simulink model "sampleModel1717"  (R2023a)
settings: Solver=VariableStepAuto  StartTime=0.0  StopTime=10.0  RelTol=1e-3
libraries: hdlsllib x4, simulink x2
settings Model: Creator=user1  LastModifiedBy=user1

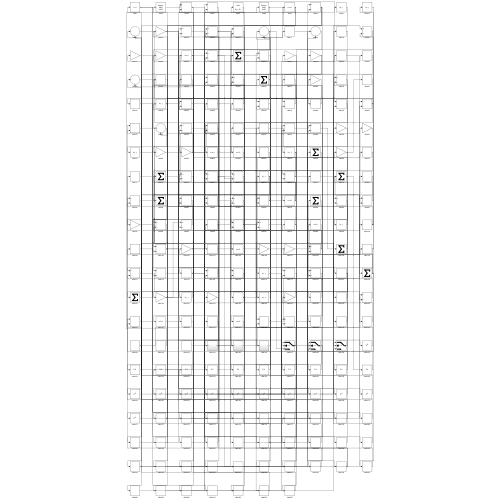
[thumbnail: Simulink's stored preview of the top-level diagram]
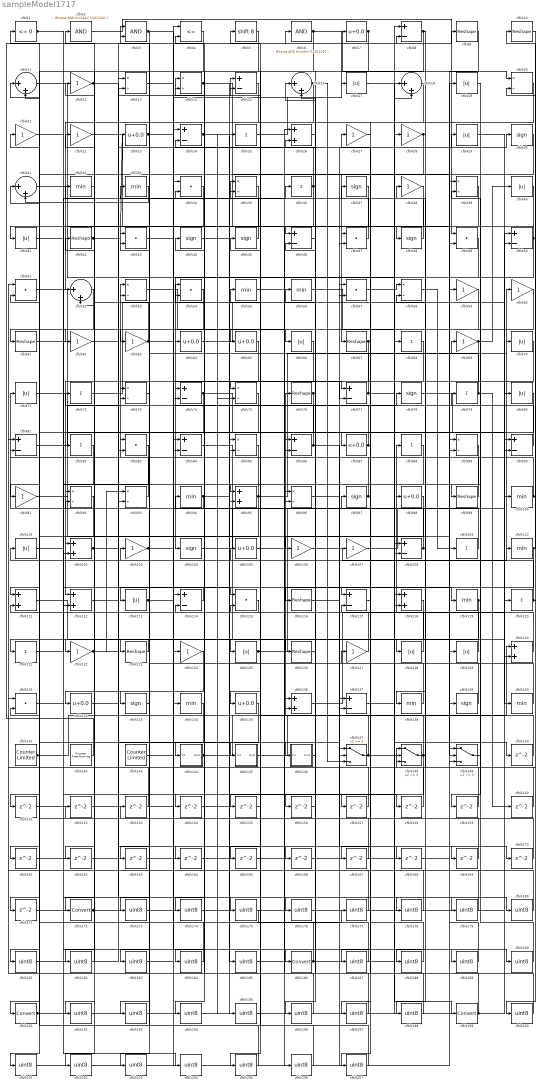
== system sampleModel1717 ==
  cfblk1 : hdlsllib/Logic and Bit Operations/Compare To Zero  relop=<=  OutDataTypeStr=boolean
  cfblk{9..10,42,61,67,76,99,116,123,126} (10 alike) : Reshape
  cfblk{32..33,55..56,94,100,110,119,134,138,140} (11 alike) : MinMax
  cfblk{17,19,29,40..41,66,70..71,80,101,113,125,128..129} (14 alike) : Abs  SaturateOnIntegerOverflow=off
  cfblk{26,95,102,111..112,118,130,136} (8 alike) : Sum
  cfblk{12,21..22,27..28,38,59..60,62..63,69,91,103,106..107,122,124,127} (18 alike) : Gain
  cfblk{30,37,44..45,48,78,97,104,133,139} (10 alike) : Signum
  cfblk{7,23,64..65,87,98,105,132,135} (9 alike) : Bias  Bias=0.0  SaturateOnIntegerOverflow=off
  cfblk{8,15,24,46,50,74,77,81,84,86,90,108,114,117,137} (15 alike) : Sum  Inputs=+-
  cfblk{25,36,68,72,79,82,88,109,120..121} (10 alike) : Sum  Inputs=+
  cfblk{11,16,18,31,52} (5 alike) : Sum  Inputs=|++
  cfblk{34,43,47,49,51,54,57,83,115,131} (10 alike) : DotProduct  OutDataTypeStr=Inherit: Inherit via internal rule
  cfblk{13..14,20,35,39,53,58,73,75,85,89,92..93,96} (14 alike) : Product  Inputs=*/  RndMeth=Zero  SaturateOnIntegerOverflow=on
  cfblk141 : hdlsllib/Sources/Counter Limited  uplimit=7  tsamp=-1
  cfblk142 : hdlsllib/Sources/Counter Free-Running  NumBits=16  tsamp=-1
  cfblk143 : hdlsllib/Sources/Counter Limited  uplimit=7  tsamp=-1
  cfblk144 : Subsystem
      settings: LibrarySourceBlock=|
      | hdlsllib/Ports &
      | Subsystems/Subsystem
  cfblk145 : Subsystem
      settings: LibrarySourceBlock=|
      | hdlsllib/Ports &
      | Subsystems/Subsystem
  cfblk146 : Subsystem
      settings: LibrarySourceBlock=|
      | hdlsllib/Ports &
      | Subsystems/Subsystem
  cfblk147 : Switch  SaturateOnIntegerOverflow=off  InputSameDT=off
  cfblk148 : Switch  SaturateOnIntegerOverflow=off  InputSameDT=off
  cfblk149 : Switch  SaturateOnIntegerOverflow=off  InputSameDT=off
  cfblk{150..171} (22 alike) : Delay  SampleTime=1
  cfblk{172,186,191,199} (4 alike) : DataTypeConversion  SaturateOnIntegerOverflow=off  RndMeth=Floor
  cfblk{173..185,187..190,192..198,200..207} (32 alike) : DataTypeConversion  OutDataTypeStr=uint8  SaturateOnIntegerOverflow=off  RndMeth=Floor
  cfblk2 : simulink/Logic and Bit Operations/Bitwise Operator  logicop=AND  UseBitMask=on  BitMask=bin2dec('11011001')  BitMaskRealWorld=Stored Integer
      settings: LibrarySourceBlock=|
      | hdlsllib/Logic and Bit
      | Operations/Bitwise
      | Operator
  cfblk3 : Logic  AllPortsSameDT=off  OutDataTypeStr=boolean
  cfblk4 : RelationalOperator  Operator=<=  OutDataTypeStr=boolean  InputSameDT=off
  cfblk5 : ArithShift  BitShiftNumber=8
  cfblk6 : simulink/Logic and Bit Operations/Bitwise Operator  logicop=AND  UseBitMask=on  BitMask=bin2dec('11011001')  BitMaskRealWorld=Stored Integer
      settings: LibrarySourceBlock=|
      | hdlsllib/Logic and Bit
      | Operations/Bitwise
      | Operator
  wires:
  cfblk58/1 -> cfblk109/1
  cfblk69/1 -> cfblk40/1, cfblk75/1
  cfblk86/1 -> cfblk53/1, cfblk158/1
  cfblk148/1 -> cfblk27/1, cfblk198/1, cfblk205/1
  cfblk109/1 -> cfblk71/1
  cfblk106/1 -> cfblk60/1
  cfblk49/1 -> cfblk104/1
  cfblk142/1 -> cfblk6/1
  cfblk66/1 -> cfblk112/1
  cfblk2/1 -> cfblk49/1
  cfblk10/1 -> cfblk148/1
  cfblk95/1 -> cfblk69/1, cfblk54/1, cfblk42/1, cfblk168/1, cfblk201/1
  cfblk28/1 -> cfblk67/1, cfblk61/1
  cfblk82/1 -> cfblk102/1
  cfblk123/1 -> cfblk121/1
  cfblk147/1 -> cfblk76/1, cfblk110/1
  cfblk128/1 -> cfblk88/1
  cfblk104/1 -> cfblk98/1
  cfblk130/1 -> cfblk37/1
  cfblk6/1 -> cfblk20/1, cfblk74/2
  cfblk51/1 -> cfblk114/1
  cfblk15/1 -> cfblk52/1
  cfblk72/1 -> cfblk50/1
  cfblk50/1 -> cfblk125/1, cfblk46/1
  cfblk114/1 -> cfblk113/1
  cfblk20/1 -> cfblk87/1
  cfblk61/1 -> cfblk84/2
  cfblk113/1 -> cfblk96/1, cfblk190/1
  cfblk65/1 -> cfblk74/1
  cfblk101/1 -> cfblk186/1
  cfblk141/1 -> cfblk130/1, cfblk1/1
  cfblk84/1 -> cfblk128/1
  cfblk32/1 -> cfblk52/2
  cfblk140/1 -> cfblk38/1
  cfblk81/1 -> cfblk73/1
  cfblk93/1 -> cfblk73/2
  cfblk22/1 -> cfblk48/1
  cfblk36/1 -> cfblk14/2, cfblk194/1
  cfblk125/1 -> cfblk97/1, cfblk155/1
  cfblk5/1 -> cfblk122/1
  cfblk59/1 -> cfblk64/1
  cfblk7/1 -> cfblk91/1, cfblk65/1
  cfblk14/1 -> cfblk89/1, cfblk146/1(In1)
  cfblk108/1 -> cfblk14/1, cfblk83/1
  cfblk30/1 -> cfblk123/1
  cfblk4/1 -> cfblk172/1
  cfblk127/1 -> cfblk5/1
  cfblk88/1 -> cfblk135/1
  cfblk60/1 -> cfblk66/1
  cfblk73/1 -> cfblk133/1
  cfblk47/1 -> cfblk35/1
  cfblk75/1 -> cfblk111/1
  cfblk34/1 -> cfblk41/1
  cfblk78/1 -> cfblk130/2
  cfblk76/1 -> cfblk132/1, cfblk174/1
  cfblk146/1(Out1) -> cfblk86/1
  cfblk27/1 -> cfblk117/1
  cfblk129/1 -> cfblk94/1
  cfblk103/1 -> cfblk78/1, cfblk9/1
  cfblk112/1 -> cfblk15/1
  cfblk110/1 -> cfblk20/2, cfblk112/2
  cfblk71/1 -> cfblk149/2
  cfblk25/1 -> cfblk7/1
  cfblk98/1 -> cfblk106/1
  cfblk11/1 -> cfblk47/1
  cfblk29/1 -> cfblk120/1
  cfblk19/1 -> cfblk99/1
  cfblk79/1 -> cfblk43/2, cfblk159/1, cfblk160/1
  cfblk137/1 -> cfblk199/1
  cfblk53/1 -> cfblk136/1
  cfblk67/1 -> cfblk77/2, cfblk187/1
  cfblk24/1 -> cfblk129/1, cfblk75/2
  cfblk149/1 -> cfblk79/1
  cfblk115/1 -> cfblk111/2
  cfblk33/1 -> cfblk31/2
  cfblk64/1 -> cfblk28/1
  cfblk136/1 -> cfblk90/1
  cfblk85/1 -> cfblk81/2
  cfblk74/1 -> cfblk118/2, cfblk83/2, cfblk195/1
  cfblk138/1 -> cfblk3/1
  cfblk105/1 -> cfblk119/1
  cfblk111/1 -> cfblk140/1
  cfblk119/1 -> cfblk171/1, cfblk203/1
  cfblk35/1 -> cfblk62/1
  cfblk77/1 -> cfblk15/2, cfblk70/1
  cfblk80/1 -> cfblk191/1
  cfblk45/1 -> cfblk24/2
  cfblk57/1 -> cfblk58/1
  cfblk42/1 -> cfblk23/1, cfblk22/1
  cfblk3/1 -> cfblk157/1, cfblk173/1
  cfblk63/1 -> cfblk17/1, cfblk32/1, cfblk77/1
  cfblk107/1 -> cfblk50/2
  cfblk122/1 -> cfblk8/2, cfblk93/1, cfblk30/1
  cfblk145/1(Out1) -> cfblk49/2
  cfblk139/1 -> cfblk105/1
  cfblk121/1 -> cfblk36/1
  cfblk94/1 -> cfblk25/1, cfblk92/2
  cfblk102/1 -> cfblk145/1(In1), cfblk166/1
  cfblk96/1 -> cfblk29/1
  cfblk83/1 -> cfblk102/2
  cfblk144/1(Out1) -> cfblk107/1, cfblk170/1
  cfblk16/1 -> cfblk63/1, cfblk93/2, cfblk147/3
  cfblk56/1 -> cfblk108/1
  cfblk62/1 -> cfblk126/1
  cfblk31/1 -> cfblk118/1
  cfblk97/1 -> cfblk44/1, cfblk197/1
  cfblk48/1 -> cfblk33/1
  cfblk87/1 -> cfblk2/1, cfblk54/2, cfblk56/1
  cfblk100/1 -> cfblk10/1, cfblk46/2
  cfblk9/1 -> cfblk89/2
  cfblk37/1 -> cfblk82/1
  cfblk99/1 -> cfblk72/1
  cfblk126/1 -> cfblk16/2
  cfblk91/1 -> cfblk139/1
  cfblk40/1 -> cfblk92/1
  cfblk38/1 -> cfblk86/2
  cfblk120/1 -> cfblk11/1, cfblk43/1, cfblk200/1
  cfblk8/1 -> cfblk95/1, cfblk138/1, cfblk116/1, cfblk144/1(In1)
  cfblk23/1 -> cfblk147/2, cfblk163/1
  cfblk12/1 -> cfblk115/1, cfblk90/2
  cfblk1/1 -> cfblk95/2, cfblk178/1
  cfblk90/1 -> cfblk3/2
  cfblk17/1 -> cfblk150/1
  cfblk150/1 -> cfblk35/2
  cfblk52/1 -> cfblk151/1
  cfblk151/1 -> cfblk24/1
  cfblk153/1 -> cfblk51/1
  cfblk41/1 -> cfblk154/1
  cfblk154/1 -> cfblk85/1
  cfblk155/1 -> cfblk115/2
  cfblk46/1 -> cfblk156/1
  cfblk156/1 -> cfblk136/2
  cfblk157/1 -> cfblk53/2
  cfblk158/1 -> cfblk148/3
  cfblk159/1 -> cfblk114/2
  cfblk160/1 -> cfblk58/2
  cfblk92/1 -> cfblk161/1
  cfblk161/1 -> cfblk149/1
  cfblk54/1 -> cfblk162/1
  cfblk162/1 -> cfblk8/1
  cfblk163/1 -> cfblk47/2
  cfblk132/1 -> cfblk164/1
  cfblk164/1 -> cfblk147/1
  cfblk89/1 -> cfblk165/1
  cfblk165/1 -> cfblk108/2
  cfblk166/1 -> cfblk96/2
  cfblk118/1 -> cfblk167/1
  cfblk167/1 -> cfblk31/1
  cfblk168/1 -> cfblk149/3
  cfblk116/1 -> cfblk169/1
  cfblk169/1 -> cfblk16/1
  cfblk170/1 -> cfblk11/2
  cfblk171/1 -> cfblk148/2
  cfblk172/1 -> cfblk152/1, cfblk19/1
  cfblk173/1 -> cfblk4/1
  cfblk174/1 -> cfblk4/2
  cfblk143/1 -> cfblk175/1
  cfblk131/1 -> cfblk176/1
  cfblk176/1 -> cfblk100/1
  cfblk175/1 -> cfblk177/1
  cfblk177/1 -> cfblk131/1
  cfblk178/1 -> cfblk131/2
  cfblk13/1 -> cfblk179/1
  cfblk179/1 -> cfblk51/2
  cfblk152/1 -> cfblk180/1
  cfblk180/1 -> cfblk13/1
  cfblk135/1 -> cfblk181/1
  cfblk181/1 -> cfblk13/2
  cfblk124/1 -> cfblk182/1
  cfblk182/1 -> cfblk12/1
  cfblk133/1 -> cfblk183/1
  cfblk183/1 -> cfblk124/1
  cfblk68/1 -> cfblk184/1
  cfblk184/1 -> cfblk153/1
  cfblk44/1 -> cfblk185/1
  cfblk185/1 -> cfblk68/1
  cfblk186/1 -> cfblk57/1, cfblk45/1
  cfblk187/1 -> cfblk101/1
  cfblk39/1 -> cfblk188/1
  cfblk188/1 -> cfblk127/1
  cfblk43/1 -> cfblk189/1
  cfblk189/1 -> cfblk39/1
  cfblk190/1 -> cfblk39/2
  cfblk191/1 -> cfblk57/2, cfblk85/2
  cfblk70/1 -> cfblk192/1
  cfblk192/1 -> cfblk80/1
  cfblk18/1 -> cfblk193/1
  cfblk193/1 -> cfblk34/1
  cfblk194/1 -> cfblk18/1
  cfblk195/1 -> cfblk18/2
  cfblk26/1 -> cfblk196/1
  cfblk196/1 -> cfblk34/2
  cfblk197/1 -> cfblk26/1
  cfblk198/1 -> cfblk26/2
  cfblk199/1 -> cfblk117/2, cfblk81/1
  cfblk200/1 -> cfblk137/1
  cfblk201/1 -> cfblk137/2
  cfblk134/1 -> cfblk202/1
  cfblk202/1 -> cfblk84/1
  cfblk203/1 -> cfblk134/1
  cfblk21/1 -> cfblk204/1
  cfblk204/1 -> cfblk59/1
  cfblk205/1 -> cfblk21/1
  cfblk55/1 -> cfblk206/1
  cfblk206/1 -> cfblk103/1
  cfblk117/1 -> cfblk207/1
  cfblk207/1 -> cfblk55/1

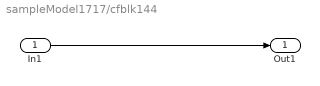
== system sampleModel1717/cfblk144 ==
  In1 : Inport
  Out1 : Outport
  wires:
  In1/1 -> Out1/1

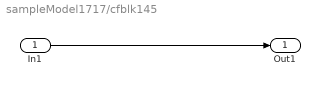
== system sampleModel1717/cfblk145 ==
  In1 : Inport
  Out1 : Outport
  wires:
  In1/1 -> Out1/1

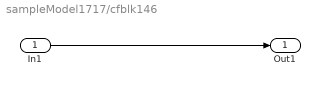
== system sampleModel1717/cfblk146 ==
  In1 : Inport
  Out1 : Outport
  wires:
  In1/1 -> Out1/1
